simulink model "final_quadruped_230622"  (R2021a)
settings: Solver=ode15s  StartTime=0.0  StopTime=10  FixedStep=1e-3  RelTol=1e-5  EnableMultiTasking=on
values from neighbouring files (symbols this model uses):
  foot_x = 8    [bipedparameters.m]    (also in fcn.m; finalrobotParameters.m; finalrobotParameters_110522.m; finalrobotParameters_140522.m)
  foot_y = 6    [bipedparameters.m]    (also in fcn.m; finalrobotParameters.m; finalrobotParameters_110522.m; finalrobotParameters_140522.m)
  foot_z = 1    [bipedparameters.m]    (also in fcn.m; finalrobotParameters.m; finalrobotParameters_110522.m; finalrobotParameters_140522.m)
  height_plane = 0.025    [bipedparameters.m]    (also in finalrobotParameters.m; finalrobotParameters_110522.m; finalrobotParameters_140522.m; finalrobotParameters_240522.m)
  kd_ankle = 1000    [bipedparameters.m]    (also in finalrobotParameters_240522.m)
  kd_hip = 1000    [bipedparameters.m]    (also in finalrobotParameters_240522.m)
  kd_knee = 1000    [bipedparameters.m]    (also in finalrobotParameters_240522.m)
  ki_ankle = 1000    [bipedparameters.m]    (also in finalrobotParameters_240522.m)
  ki_hip = 1000    [bipedparameters.m]    (also in finalrobotParameters_240522.m)
  ki_knee = 2000    [bipedparameters.m]    (also in finalrobotParameters_240522.m)
  kp_ankle = 1000    [bipedparameters.m]    (also in finalrobotParameters_240522.m)
  kp_hip = 1000    [bipedparameters.m]    (also in finalrobotParameters_240522.m)
  kp_knee = 2000    [bipedparameters.m]    (also in finalrobotParameters_240522.m)
  lower_leg_length = 10    [bipedparameters.m]    (also in fcn.m; finalrobotParameters.m; finalrobotParameters_110522.m; finalrobotParameters_140522.m)
  plane_x = 25    [bipedparameters.m]    (also in finalrobotParameters.m; finalrobotParameters_110522.m; finalrobotParameters_140522.m; finalrobotParameters_240522.m)
  plane_y = 3    [bipedparameters.m]    (also in finalrobotParameters.m; finalrobotParameters_110522.m; finalrobotParameters_140522.m; finalrobotParameters_240522.m)
  torso_offset_x = -0.5    [bipedparameters.m]    (also in finalrobotParameters.m = 10; finalrobotParameters_110522.m = 10; finalrobotParameters_140522.m = 10; finalrobotParameters_240522.m = 10)
  torso_offset_z = -2    [bipedparameters.m]    (also in finalrobotParameters.m; finalrobotParameters_110522.m; finalrobotParameters_140522.m; finalrobotParameters_240522.m)
  torso_x = 5    [bipedparameters.m]    (also in fcn.m = 25; finalrobotParameters.m = 25; finalrobotParameters_110522.m = 25; finalrobotParameters_140522.m = 25)
  torso_y = 10    [bipedparameters.m]    (also in fcn.m = 16; finalrobotParameters.m = 16; finalrobotParameters_110522.m = 16; finalrobotParameters_140522.m = 16)
  torso_z = 8    [bipedparameters.m]    (also in fcn.m = 10; finalrobotParameters.m = 10; finalrobotParameters_110522.m = 10; finalrobotParameters_140522.m = 10)
  upper_leg_length = 10    [bipedparameters.m]    (also in fcn.m; finalrobotParameters.m; finalrobotParameters_110522.m; finalrobotParameters_140522.m)
undefined symbols (not defined in the file or in its folder): sigbuilder_block, X, Y, Z
libraries: nesl_utility x246, sm_lib x71, pid_lib x20, Contact_Forces_Lib x16, fl_lib x4
(part 1 of 8)
settings Model: Creator=Durbadal Guest  LastModifiedBy=Saniya
settings DataIOCC: LimitDataPoints=on  SaveFormat=StructureWithTime  ReturnWorkspaceOutputs=off
settings OptimizationCC: LifeSpan=inf
settings DebuggingCC: SFUnexpectedBacktrackingDiag=warning  SFNoUnconditionalDefaultTransitionDiag=warning  SFExecutionAtInitializationDiag=none  SFMachineParentedDataDiag=warning  ArithmeticOperatorsInVariantConditions=warning
settings HardwareCC: ProdBitPerSizeT=32  ProdBitPerPtrDiffT=32  ProdWordSize=32  ProdHWDeviceType=Specified
settings SFSimCC: SimUseLocalCustomCode=off  CustomCodeUndefinedFunction=UseInterfaceOnly
settings RTWCC: RTWUseLocalCustomCode=off
settings CodeAppCC: StateflowObjectComments=on
settings GRTTargetCC: TargetLangStandard=C89/C90 (ANSI)
settings ConfigComp: CovMetricSettings=dw  CovSaveCumulativeToWorkspaceVar=on  CovSaveSingleToWorkspaceVar=on  CovExternalEMLEnable=off  CovSFcnEnable=off
settings SimscapeCC: SimscapeNominalValues="[{\"value\":\"10\",\"unit\":\"V\"},{\"value\":\"1\",\"unit\":\"A\"},{\"value\":\"10\",\"unit\":\"N*m\"},{\"value\":\"10\",\"unit\":\"bar\"},{\"value\":\"100\",\"unit\":\"kJ/kg\"},{\"value\":\"1\",\"unit\":\"kW\"},{\"value\":\"300\",\"unit\":\"K\"},{\"value\":\"100\",\"unit\":\"cm^3/s\"},{\"value\":\"1\",\"unit\":\"kN\"},{\"value\":\"1\",\"unit\":\"g/cm^3\"},{\"value\":\"1\",\"unit\":\"l\"},{\"value\":\"1\",\"unit\":\"cm^2\"},{\"value\":\"60\",\"unit\":\"Hz\"}]"  SimscapeLogType=all  SimscapeLogDataHistory=10000
settings ConfigurationSet: Description=SimMechanics 2G
settings DiagnosticsConfigSet: SimMechanicsRigidlyBoundBlock=none

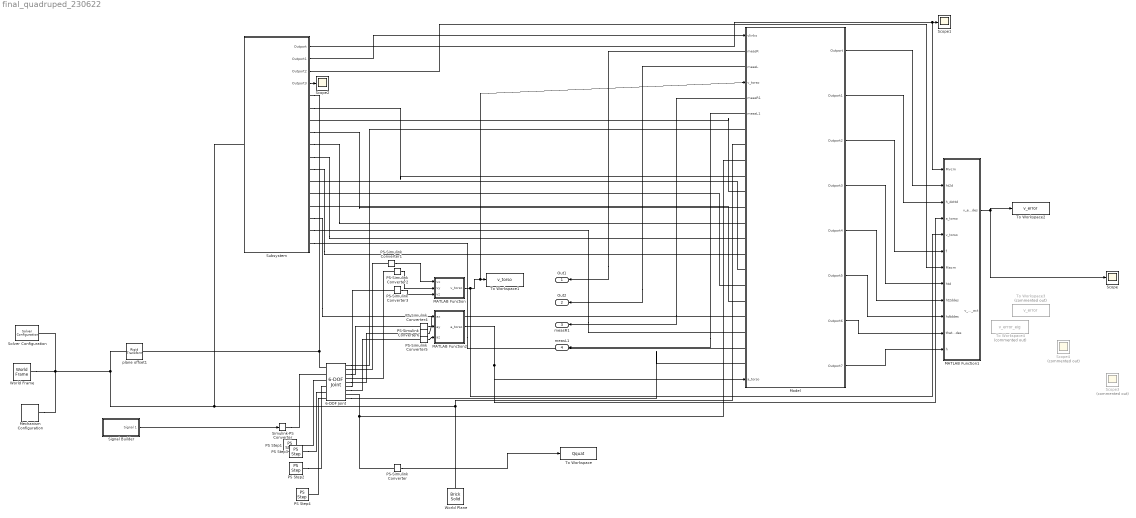
== system final_quadruped_230622 ==
  6-DOF Joint : sm_lib/Joints/6-DOF Joint  JointMode=Normal  SenseConstraintForce=off  SenseConstraintForceX=off  SenseConstraintForceY=off  SenseConstraintForceZ=off  SenseConstraintTorque=off  SenseConstraintTorqueX=off  SenseConstraintTorqueY=off  SenseConstraintTorqueZ=off  SenseTotalForce=off  SenseTotalForceX=off  SenseTotalForceY=off  SenseTotalForceZ=off  SenseTotalTorque=off  SenseTotalTorqueX=off  SenseTotalTorqueY=off  SenseTotalTorqueZ=off  CompositeWrenchDir=FollowerOnBase  CompositeWrenchFrame=BaseFrame  PxEquilibriumPosition=0  PxEquilibriumPositionUnits=m  PxSpringStiffness=0  PxSpringStiffnessUnits=N/m  PxDampingCoefficient=0  PxDampingCoefficientUnits=N/(m/s)  PxTorqueActuationMode=InputTorque  PxMotionActuationMode=ComputedMotion  PxSensePosition=off  PxSenseVelocity=on  PxSenseAcceleration=on  PxSenseTorqueForce=off  PxSenseLowerLimitTorqueForce=off  PxSenseUpperLimitTorqueForce=off  PxLowerLimitSpecify=off  PxLowerLimitBound=-1  PxLowerLimitBoundUnits=m  PxLowerLimitStiffness=1e6  PxLowerLimitStiffnessUnits=N/m  PxLowerLimitDamping=1e3  PxLowerLimitDampingUnits=N/(m/s)  PxLowerLimitTransitionRegionWidth=1e-4  PxLowerLimitTransitionRegionWidthUnits=m  PxUpperLimitSpecify=off  PxUpperLimitBound=1  PxUpperLimitBoundUnits=m  PxUpperLimitStiffness=1e6  PxUpperLimitStiffnessUnits=N/m  PxUpperLimitDamping=1e3  PxUpperLimitDampingUnits=N/(m/s)  PxUpperLimitTransitionRegionWidth=1e-4  PxUpperLimitTransitionRegionWidthUnits=m  PxPositionTargetSpecify=on  PxPositionTargetPriority=High  PxPositionTargetValue=0  PxPositionTargetValueUnits=m  PxVelocityTargetSpecify=off  PxVelocityTargetPriority=High  PxVelocityTargetValue=0  PxVelocityTargetValueUnits=m/s  PyEquilibriumPosition=0  PyEquilibriumPositionUnits=m  PySpringStiffness=0  PySpringStiffnessUnits=N/m  PyDampingCoefficient=0  PyDampingCoefficientUnits=N/(m/s)  PyTorqueActuationMode=InputTorque  PyMotionActuationMode=ComputedMotion  PySensePosition=off  PySenseVelocity=on  PySenseAcceleration=on  PySenseTorqueForce=off  PySenseLowerLimitTorqueForce=off  PySenseUpperLimitTorqueForce=off  PyLowerLimitSpecify=off  PyLowerLimitBound=-1  PyLowerLimitBoundUnits=m  PyLowerLimitStiffness=1e6  PyLowerLimitStiffnessUnits=N/m  PyLowerLimitDamping=1e3  PyLowerLimitDampingUnits=N/(m/s)  PyLowerLimitTransitionRegionWidth=1e-4  PyLowerLimitTransitionRegionWidthUnits=m  PyUpperLimitSpecify=off  PyUpperLimitBound=1  PyUpperLimitBoundUnits=m  PyUpperLimitStiffness=1e6  PyUpperLimitStiffnessUnits=N/m  PyUpperLimitDamping=1e3  PyUpperLimitDampingUnits=N/(m/s)  PyUpperLimitTransitionRegionWidth=1e-4  PyUpperLimitTransitionRegionWidthUnits=m  PyPositionTargetSpecify=on  PyPositionTargetPriority=High  PyPositionTargetValue=0  PyPositionTargetValueUnits=m  PyVelocityTargetSpecify=off  PyVelocityTargetPriority=High  PyVelocityTargetValue=0  PyVelocityTargetValueUnits=m/s  PzEquilibriumPosition=0  PzEquilibriumPositionUnits=m  PzSpringStiffness=0  PzSpringStiffnessUnits=N/m  PzDampingCoefficient=0  PzDampingCoefficientUnits=N/(m/s)  PzTorqueActuationMode=InputTorque  PzMotionActuationMode=ComputedMotion  PzSensePosition=off  PzSenseVelocity=on  PzSenseAcceleration=on  PzSenseTorqueForce=off  PzSenseLowerLimitTorqueForce=off  PzSenseUpperLimitTorqueForce=off  PzLowerLimitSpecify=off  PzLowerLimitBound=-1  PzLowerLimitBoundUnits=m  PzLowerLimitStiffness=1e6  PzLowerLimitStiffnessUnits=N/m  PzLowerLimitDamping=1e3  PzLowerLimitDampingUnits=N/(m/s)  PzLowerLimitTransitionRegionWidth=1e-4  PzLowerLimitTransitionRegionWidthUnits=m  PzUpperLimitSpecify=off  PzUpperLimitBound=1  PzUpperLimitBoundUnits=m  PzUpperLimitStiffness=1e6  PzUpperLimitStiffnessUnits=N/m  PzUpperLimitDamping=1e3  PzUpperLimitDampingUnits=N/(m/s)  PzUpperLimitTransitionRegionWidth=1e-4  PzUpperLimitTransitionRegionWidthUnits=m  PzPositionTargetSpecify=on  PzPositionTargetPriority=High  PzPositionTargetValue=0  PzPositionTargetValueUnits=m  PzVelocityTargetSpecify=off  PzVelocityTargetPriority=High  PzVelocityTargetValue=0  PzVelocityTargetValueUnits=m/s  SphDefPosRotationMethod=None  SphDefPosRotationAngleUnits=deg  SphDefPosRotationStandardAxis=+Z  SphDefPosRotationAngle=0.0  SphDefPosRotationArbitraryAxis=[0 0 1]  SphDefPosFollAlignAxisA=+X  SphDefPosBaseAlignAxisA=+Y  SphDefPosFollAlignAxisB=+Y  SphDefPosBaseAlignAxisB=+Z  SphDefPosRotationSequenceAxes=FollowerAxes  SphDefPosRotationSequence=XYX  SphDefPosRotationSequenceAngles=[0 0 0]  SphDefPosRotationSequenceAnglesUnits=deg  SphDefPosRotationMatrix=[1 0 0; 0 1 0; 0 0 1]  SphEqPosRotationMethod=None  SphEqPosRotationAngleUnits=deg  SphEqPosRotationStandardAxis=+Z  SphEqPosRotationAngle=0.0  SphEqPosRotationArbitraryAxis=[0 0 1]  SphEqPosFollAlignAxisA=+X  SphEqPosBaseAlignAxisA=+Y  SphEqPosFollAlignAxisB=+Y  SphEqPosBaseAlignAxisB=+Z  SphEqPosRotationSequenceAxes=FollowerAxes  SphEqPosRotationSequence=XYX  SphEqPosRotationSequenceAngles=[0 0 0]  SphEqPosRotationSequenceAnglesUnits=deg  SphEqPosRotationMatrix=[1 0 0; 0 1 0; 0 0 1]  SphSpringStiffness=0  SphSpringStiffnessUnits=N*m/deg  SphDampingCoefficient=world_rot_damping  SphDampingCoefficientUnits=N*m/(deg/s)  SphActuateTorqueX=on  SphActuateTorqueY=off  SphActuateTorqueZ=on  SphActuateTorque=off  SphTorqueActuationMode=InputTorque  SphMotionActuationMode=ComputedMotion  SphActuationFrame=BaseFrame  SphSensePosition=on  SphSenseVelocityX=off  SphSenseVelocityY=off  SphSenseVelocityZ=off  SphSenseVelocity=on  SphSenseAccelerationX=off  SphSenseAccelerationY=off  SphSenseAccelerationZ=off  SphSenseAcceleration=off  SphSenseTorqueX=off  SphSenseTorqueY=off  SphSenseTorqueZ=off  SphSenseTorqueForce=off  SphSenseLowerLimitTorqueMag=off  SphSenseUpperLimitTorqueMag=off  SphSensingFrame=BaseFrame  SphLowerLimitSpecify=off  SphLowerLimitBound=15  SphLowerLimitBoundUnits=deg  SphLowerLimitStiffness=1e4  SphLowerLimitStiffnessUnits=N*m/deg  SphLowerLimitDamping=10  SphLowerLimitDampingUnits=N*m/(deg/s)  SphLowerLimitTransitionRegionWidth=0.1  SphLowerLimitTransitionRegionWidthUnits=deg  SphUpperLimitSpecify=off  SphUpperLimitBound=45  SphUpperLimitBoundUnits=deg  SphUpperLimitStiffness=1e4  SphUpperLimitStiffnessUnits=N*m/deg  SphUpperLimitDamping=10  SphUpperLimitDampingUnits=N*m/(deg/s)  SphUpperLimitTransitionRegionWidth=0.1  SphUpperLimitTransitionRegionWidthUnits=deg  SphPositionTargetRotationMethod=None  SphPositionTargetRotationAngleUnits=deg  SphPositionTargetRotationStandardAxis=+Z  SphPositionTargetRotationAngle=0.0  SphPositionTargetRotationArbitraryAxis=[0 0 1]  SphPositionTargetFollAlignAxisA=+X  SphPositionTargetBaseAlignAxisA=+Y  SphPositionTargetFollAlignAxisB=+Y  SphPositionTargetBaseAlignAxisB=+Z  SphPositionTargetRotationSequenceAxes=FollowerAxes  SphPositionTargetRotationSequence=XYX  SphPositionTargetRotationSequenceAngles=[0 0 0]  SphPositionTargetRotationSequenceAnglesUnits=deg  SphPositionTargetRotationMatrix=[1 0 0; 0 1 0; 0 0 1]  SphPositionTargetSpecify=off  SphPositionTargetPriority=High  SphVelocityTargetValue=[0 0 0]  SphVelocityTargetValueUnits=deg/s  SphVelocityTargetSpecify=off  SphVelocityTargetPriority=High  SphVelocityTargetInFollowerFrame=on
  MATLAB Function : MATLAB Function  TreatAsAtomicUnit=on
  MATLAB Function1 : MATLAB Function  TreatAsAtomicUnit=on
  MATLAB Function2 : MATLAB Function  TreatAsAtomicUnit=on
  Mechanism Configuration : sm_lib/Utilities/Mechanism Configuration  UniformGravity=Constant  GravityVector=[0 0 -9.80665]  GravityVectorUnits=m/s^2  GravityUnits=m/s^2  LinearizationDelta=0.001  JointModeTransitionNonlinearIterations=2
  Model : Subsystem
      settings: PortSchema="{\"entries\":[{\"content\":{\"sides\":[{\"content\":{\"connectorIds\":[\"Out5\",\"Out6\",\"Out7\",\"Out8\",\"Out9\",\"Out10\",\"Out11\",\"Out12\"]},\"type\":\"ConnectorPlacement.EquallySpacedRectSide\",\"uuid\":\"648e0f1c-94fd-432d-b314-f859853b28dc\"},{\"content\":{\"connectorIds\":[\"In1\",\"Out1\",\"Out2\",\"In2\",\"Out3\",\"Out4\",\"RConn1\",\"RConn2\",\"RConn3\",\"RConn4\",\"RConn5\",\"RConn6\",\"RConn7\",\"RConn8\",\"RConn9\",\"RConn10\",\"RConn11\",\"RConn12\",\"RConn13\",\"RConn14\",\"RConn15\",\"RConn16\",\"In3\"],\"side\":\"RIGHT\"},\"type\":\"ConnectorPlacement.EquallySpacedRectSide\",\"uuid\":\"4a085109-6c7b-452e-9c34-33db191f9143\"},{\"content\":{\"connectorIds\":[],\"side\":\"TOP\"},\"type\":\"ConnectorPlacement.EquallySpacedRectSide\",\"uuid\":\"a578f37e-fb06-4d5d-8e21-8bc1ba433708\"},{\"content\":{\"connectorIds\":[],\"side\":\"BOTTOM\"},\"type\":\"ConnectorPlacement.EquallySpacedRectSide\",\"uuid\":\"167a25d4-eaf5-4df2-a71c-c676bae0267f\"}]},\"type\":\"ConnectorPlacement.EquallySpacedConnector\",\"uuid\":\"512c293d-fddc-4597-a716-0ff05cc0aa2f\"}],\"packageUris\":[\"http://schema.mathworks.com/mf0/Connector/R2020b\"],\"version\":\"1.0\"}"
  PS Step1 : fl_lib/Physical Signals/Sources/PS Step  step_time=0 s  initial_value=0 N  final_value=0 N
      settings: SourceProductBaseCode=SS
  PS Step2 : fl_lib/Physical Signals/Sources/PS Step  step_time=1 s  initial_value=0 N  final_value=0 N
      settings: SourceProductBaseCode=SS
  PS Step3 : fl_lib/Physical Signals/Sources/PS Step  step_time=1 s  initial_value=0 N*m  final_value=0 N*m
      settings: SourceProductBaseCode=SS
  PS Step4 : fl_lib/Physical Signals/Sources/PS Step  step_time=0 s  initial_value=0 N*m  final_value=1 N*m
      settings: SourceProductBaseCode=SS
  PS-Simulink Converter{,1..6} (7 alike) : nesl_utility/PS-Simulink Converter  PhysicalDomain=network_engine_domain  SubClassName=ps_output  LeftPortType=input  RightPortType=output  PseudoPeriodic=off  Frequencies=[]  Unit=inherit  AffineConversion=off
      settings: SourceProductBaseCode=PW,SS
  Scope : Scope
  Scope1 : Scope
  Scope2 : Scope
  Scope3 : Scope  Commented=on
  Scope4 : Scope  Commented=on
  Signal Builder : Subsystem  Tag=STV Subsys  LoadFcn=sigbuilder_block('load');  StartFcn=sigbuilder_block('start');  StopFcn=sigbuilder_block('stop');  ClipboardFcn=sigbuilder_block('clipboard');  mask(Sigbuilder block){tuvar=[0:10]}
      mask help: Simulink:masks:SigbuilderBlock_MD
      mask init:
      | if ~strcmp(get_param(bdroot(gcbh),'SimulationStatus'),'stopped') tuvar = sigbuilder_block('maskInit'); end
      settings: CopyFcn=sigbuilder_block('copy');  DeleteFcn=sigbuilder_block('delete');  ModelCloseFcn=sigbuilder_block('modelClose');  PreSaveFcn=sigbuilder_block('preSave');  PauseFcn=sigbuilder_block('pause');  ContinueFcn=sigbuilder_block('continue');  NameChangeFcn=sigbuilder_block('namechange');  OpenFcn=sigbuilder_block('open',[5.5 36 949 412 ]);  CloseFcn=sigbuilder_block('close');
      mask Display: plot(0, 0, 100, 100,[2, 2, 32, 32, 2], [68, 8, 8, 68, 68],[32, 2], [38, 38], [32, 19, 2],[53, 60, 44], [32, 17, 17, 2],[16, 16, 31, 31]);txt = getActiveGroup(gcbh);text(2, 100, txt,'verticalAlignment', 'top');
  Simulink-PS Converter : nesl_utility/Simulink-PS Converter  PhysicalDomain=network_engine_domain  SubClassName=ps_input  LeftPortType=input  RightPortType=output  PseudoPeriodic=off  Frequencies=[]  NoiseDistribution=none  NoiseParameters=[]  Unit=1  AffineConversion=off  FilteringAndDerivatives=provide  SimscapeFilterOrder=1  InputFilterTimeConstant=0.001  UdotUserProvided=0
      settings: SourceProductBaseCode=PW,SS
  Solver Configuration : nesl_utility/Solver Configuration  PhysicalDomain=network_engine_domain  SubClassName=solver  LeftPortType=input  RightPortType=generic  Tones=[]  Harmonics=[]  SimulateNoise=off  Profile=off  UseLocalSampling=off  EnableSwitchedLinearOptims=on  FrequencyDomain=off  UseCCode=off  RelTol=0.001  AbsTol=1e-06  MinStep=1e-09  ToWorkspace=off  RevertToSquareIcSolve=off  NumHomotopyIterations=100  PhasorMode=off  PhasorModeNumHarmonics=1  DoDC=off  ResidualTolerance=1e-09  UseLocalSolver=off  LocalSolverChoice=NE_BACKWARD_EULER_ADVANCER  LocalSolverSampleTime=0.001  DoFixedCost=off  MaxNonlinIter=3  MaxModeIter=2  ComputeImpulses=off  ImpulseIterations=2  LinearAlgebra=Full  EquationFormulation=NE_TIME_EF  DelaysMemoryBudget=1024  AutomaticFiltering=on  FilteringTimeConstant=0.001  PartitionStorageMethod=AS_NEEDED  PartitionMemoryBudget=1024  PartitionMethod=FAST
      settings: SourceProductBaseCode=PW,SS
  Subsystem : Subsystem
  To Workspace : ToWorkspace  VariableName=Qquat  SaveFormat=Timeseries  SampleTime=-1
  To Workspace1 : ToWorkspace  VariableName=v_torso  SaveFormat=Timeseries  SampleTime=-1
  To Workspace2 : ToWorkspace  VariableName=v_error  SaveFormat=Timeseries  SampleTime=-1
  To Workspace3 : ToWorkspace  Commented=on  VariableName=v_error  SaveFormat=Timeseries  SampleTime=-1
  To Workspace4 : ToWorkspace  Commented=on  VariableName=v_error_eig  SaveFormat=Timeseries  SampleTime=-1
  World Frame : sm_lib/Frames and Transforms/World Frame
  World Plane : sm_lib/Body Elements/Brick Solid  GraphicAmbientColor=[0.15 0.15 0.15 1.0]  BasedOnType=Density  BrickDimensions=[plane_x plane_y height_plane]  BrickDimensionUnits=m  CenterOfMass=[0 0 0]  CenterOfMassUnits=m  GraphicDiffuseColor=[1.0 0.2 0.2]  Density=2000  DensityUnits=kg/m^3  DoExposeReferenceFrame=on  GraphicEmissiveColor=[0.0 0.0 0.0 1.0]  ExportEntireGeometry=off  SerializedFrames=<Frames/>  MarkerShape=Sphere  MarkerSize=10  GraphicType=FromGeometry  InertiaType=CalculateFromGeometry  Mass=1  MassUnits=kg  MomentsOfInertia=[1 1 1]  MomentsOfInertiaUnits=kg*m^2  GraphicOpacity=1.0  ProductsOfInertia=[1 1 1]  ProductsOfInertiaUnits=kg*m^2  GraphicShininess=75  GraphicSpecularColor=[0.5 0.5 0.5 1.0]  GraphicVisPropType=SimpleVisualProperties
  plane offset1 : sm_lib/Frames and Transforms/Rigid Transform  TranslationMethod=StandardAxis  TranslationStandardOffset=24.1  TranslationLengthUnit=cm  TranslationStandardAxis=+Z  TranslationCartesianOffset=[0 0 0]  TranslationROffset=0  TranslationROffsetUnits=m  TranslationZOffset=0  TranslationZOffsetUnits=m  TranslationThetaOffset=0  TranslationThetaOffsetUnits=deg  RotationMethod=None  RotationAngleUnits=deg  RotationStandardAxis=+Z  RotationAngle=0.0  RotationArbitraryAxis=[0 0 1]  FollAlignAxisA=+X  BaseAlignAxisA=+Y  FollAlignAxisB=+Y  BaseAlignAxisB=+Z  RotationSequenceAxes=FollowerAxes  RotationSequence=XYX  RotationSequenceAngles=[0 0 0]  RotationSequenceAnglesUnits=deg  RotationMatrix=[1 0 0; 0 1 0; 0 0 1]
  Out1 : Outport  VectorParamsAs1DForOutWhenUnconnected=off
  Out2 : Outport  Port=2  VectorParamsAs1DForOutWhenUnconnected=off
  measR1 : Outport  Port=3  VectorParamsAs1DForOutWhenUnconnected=off
  measL1 : Outport  Port=4  VectorParamsAs1DForOutWhenUnconnected=off
  wires:
  Model/1(measR) -> Out1/1
  Model/2(measL) -> Out2/1
  Model/3(measR1) -> measR1/1
  Model/4(measL1) -> measL1/1
  PS-Simulink Converter/1 -> To Workspace/1
  PS-Simulink Converter1/1 -> MATLAB Function/1(vx)
  PS-Simulink Converter2/1 -> MATLAB Function/2(vy)
  PS-Simulink Converter3/1 -> MATLAB Function/3(vz)
  Subsystem/1(Outport) -> Scope1/1, MATLAB Function1/1(Mvcm)
  Model/5(Outport) -> MATLAB Function1/2(ht2d)
  MATLAB Function/1(v_torso) -> MATLAB Function1/5(v_torso), To Workspace1/1, Model/2(v_torso)
  Subsystem/2(Outport1) -> Model/1(vlinks)
  PS-Simulink Converter4/1 -> MATLAB Function2/1(ax)
  PS-Simulink Converter5/1 -> MATLAB Function2/3(az)
  PS-Simulink Converter6/1 -> MATLAB Function2/2(ay)
  MATLAB Function2/1(a_torso) -> MATLAB Function1/4(a_torso), Model/3(a_torso)
  Model/6(Outport1) -> MATLAB Function1/3(h_dottd)
  Model/7(Outport2) -> MATLAB Function1/6(f)
  Subsystem/3(Outport2) -> MATLAB Function1/7(Macm)
  Subsystem/4(Outport3) -> Scope2/1
  Model/8(Outport3) -> MATLAB Function1/8(htd)
  MATLAB Function1/1(v_error_des) -> Scope/1, To Workspace2/1
  Model/9(Outport4) -> MATLAB Function1/9(ht2ddes)
  Model/10(Outport5) -> MATLAB Function1/10(hdtddes)
  ? -> Scope3/1, To Workspace3/1
  Model/11(Outport6) -> MATLAB Function1/11(theta_d_des)
  Model/12(Outport7) -> MATLAB Function1/12(h)
  ? -> Scope4/1, To Workspace4/1
  Signal Builder/1(Signal 1) -> Simulink-PS Converter/1
  connections:
  6-DOF Joint/RConn1 -- Model/RConn1
  6-DOF Joint/LConn1 -- plane offset1/RConn1 -- Subsystem/RConn1
  PS-Simulink Converter/LConn1 -- 6-DOF Joint/RConn8 -- Model/RConn3
  PS-Simulink Converter1/LConn1 -- 6-DOF Joint/RConn2
  PS-Simulink Converter2/LConn1 -- 6-DOF Joint/RConn4
  plane offset1/LConn1 -- Solver Configuration/RConn1 -- World Frame/RConn1 -- Mechanism Configuration/RConn1 -- Subsystem/LConn1 -- World Plane/RConn1 -- Model/RConn2
  Subsystem/RConn2 -- Model/RConn4
  Model/RConn5 -- Subsystem/RConn3
  Subsystem/RConn4 -- Model/RConn6
  Subsystem/RConn5 -- Model/RConn7
  Subsystem/RConn6 -- Model/RConn8
  Subsystem/RConn7 -- Model/RConn9
  Model/RConn10 -- Subsystem/RConn8
  Model/RConn11 -- Subsystem/RConn9
  Model/RConn12 -- Subsystem/RConn10
  Subsystem/RConn11 -- Model/RConn13
  Subsystem/RConn12 -- Model/RConn14
  Subsystem/RConn13 -- Model/RConn15
  PS Step1/RConn1 -- 6-DOF Joint/LConn3
  PS Step2/RConn1 -- 6-DOF Joint/LConn4
  PS Step3/RConn1 -- 6-DOF Joint/LConn5
  6-DOF Joint/RConn9 -- Model/RConn16
  6-DOF Joint/RConn6 -- PS-Simulink Converter3/LConn1
  6-DOF Joint/RConn3 -- PS-Simulink Converter4/LConn1
  6-DOF Joint/RConn5 -- PS-Simulink Converter6/LConn1
  6-DOF Joint/RConn7 -- PS-Simulink Converter5/LConn1
  Simulink-PS Converter/RConn1 -- 6-DOF Joint/LConn2
  6-DOF Joint/LConn6 -- PS Step4/RConn1

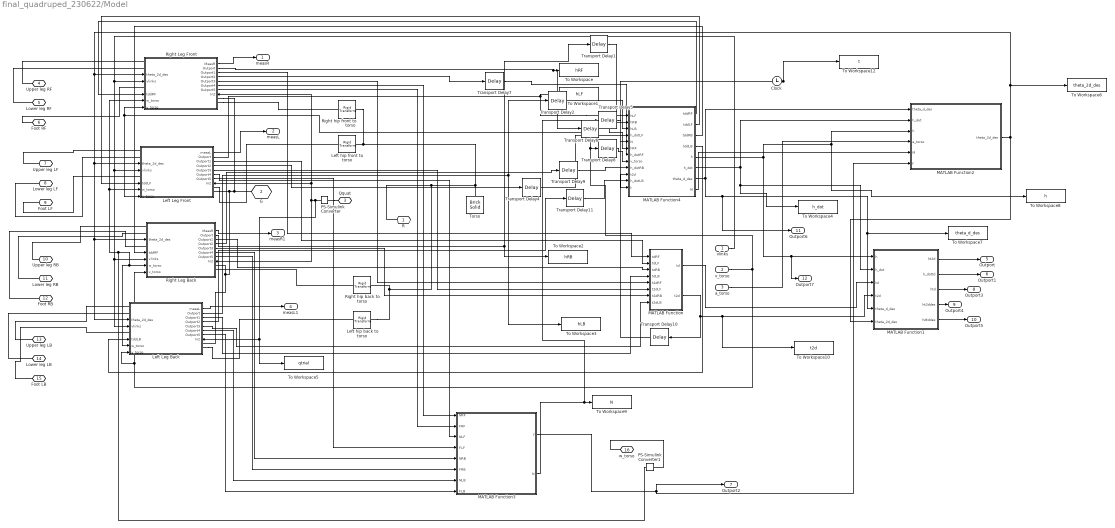
== system final_quadruped_230622/Model ==
  vlinks : Inport
  v_torso : Inport  Port=2
  a_torso : Inport  Port=3
  Clock : Clock
  Left Leg Back : Subsystem
      settings: PortSchema="{\"entries\":[{\"content\":{\"sides\":[{\"content\":{\"connectorIds\":[\"LConn1\",\"LConn2\",\"In1\",\"In2\",\"LConn3\",\"In3\",\"In4\",\"In5\"]},\"type\":\"ConnectorPlacement.EquallySpacedRectSide\",\"uuid\":\"22ee734e-d516-4767-9dd7-a84a6d7499a1\"},{\"content\":{\"connectorIds\":[\"Out1\",\"Out2\",\"Out3\",\"Out4\",\"Out5\",\"Out6\",\"Out7\",\"In6\",\"RConn1\",\"RConn2\"],\"side\":\"RIGHT\"},\"type\":\"ConnectorPlacement.EquallySpacedRectSide\",\"uuid\":\"10c942f7-94ea-46a3-ba7f-65e81ae36ff4\"},{\"content\":{\"connectorIds\":[],\"side\":\"TOP\"},\"type\":\"ConnectorPlacement.EquallySpacedRectSide\",\"uuid\":\"f15406a8-c456-4a24-8e06-fd295582a32c\"}]},\"type\":\"ConnectorPlacement.EquallySpacedConnector\",\"uuid\":\"8882591f-f267-4868-b883-a2707b6c50ed\"}],\"packageUris\":[\"http://schema.mathworks.com/mf0/Connector/R2020b\"],\"version\":\"1.0\"}"
  "Left Leg Front " : Subsystem
      settings: PortSchema="{\"entries\":[{\"content\":{\"sides\":[{\"content\":{\"connectorIds\":[\"LConn1\",\"LConn2\",\"In1\",\"In2\",\"LConn3\",\"In3\",\"In4\",\"In5\"]},\"type\":\"ConnectorPlacement.EquallySpacedRectSide\",\"uuid\":\"22ee734e-d516-4767-9dd7-a84a6d7499a1\"},{\"content\":{\"connectorIds\":[\"Out1\",\"Out2\",\"Out3\",\"Out4\",\"Out5\",\"Out6\",\"Out7\",\"In6\",\"RConn1\",\"RConn2\"],\"side\":\"RIGHT\"},\"type\":\"ConnectorPlacement.EquallySpacedRectSide\",\"uuid\":\"10c942f7-94ea-46a3-ba7f-65e81ae36ff4\"},{\"content\":{\"connectorIds\":[],\"side\":\"TOP\"},\"type\":\"ConnectorPlacement.EquallySpacedRectSide\",\"uuid\":\"f15406a8-c456-4a24-8e06-fd295582a32c\"}]},\"type\":\"ConnectorPlacement.EquallySpacedConnector\",\"uuid\":\"8882591f-f267-4868-b883-a2707b6c50ed\"}],\"packageUris\":[\"http://schema.mathworks.com/mf0/Connector/R2020b\"],\"version\":\"1.0\"}"
  Left hip back to torso : sm_lib/Frames and Transforms/Rigid Transform  TranslationMethod=Cartesian  TranslationStandardOffset=0  TranslationLengthUnit=cm  TranslationStandardAxis=+Z  TranslationCartesianOffset=[-torso_offset_x torso_y/2 torso_offset_z]  TranslationROffset=0  TranslationROffsetUnits=m  TranslationZOffset=0  TranslationZOffsetUnits=m  TranslationThetaOffset=0  TranslationThetaOffsetUnits=deg  RotationMethod=None  RotationAngleUnits=deg  RotationStandardAxis=+Z  RotationAngle=0.0  RotationArbitraryAxis=[0 0 1]  FollAlignAxisA=+X  BaseAlignAxisA=+Y  FollAlignAxisB=+Y  BaseAlignAxisB=+Z  RotationSequenceAxes=FollowerAxes  RotationSequence=XYX  RotationSequenceAngles=[0 0 0]  RotationSequenceAnglesUnits=deg  RotationMatrix=[1 0 0; 0 1 0; 0 0 1]
  Left hip front to torso : sm_lib/Frames and Transforms/Rigid Transform  TranslationMethod=Cartesian  TranslationStandardOffset=0  TranslationLengthUnit=cm  TranslationStandardAxis=+Z  TranslationCartesianOffset=[torso_offset_x torso_y/2 torso_offset_z]  TranslationROffset=0  TranslationROffsetUnits=m  TranslationZOffset=0  TranslationZOffsetUnits=m  TranslationThetaOffset=0  TranslationThetaOffsetUnits=deg  RotationMethod=None  RotationAngleUnits=deg  RotationStandardAxis=+Z  RotationAngle=0.0  RotationArbitraryAxis=[0 0 1]  FollAlignAxisA=+X  BaseAlignAxisA=+Y  FollAlignAxisB=+Y  BaseAlignAxisB=+Z  RotationSequenceAxes=FollowerAxes  RotationSequence=XYX  RotationSequenceAngles=[0 0 0]  RotationSequenceAnglesUnits=deg  RotationMatrix=[1 0 0; 0 1 0; 0 0 1]
  MATLAB Function : MATLAB Function  TreatAsAtomicUnit=on
  MATLAB Function1 : MATLAB Function  TreatAsAtomicUnit=on
  MATLAB Function2 : MATLAB Function  TreatAsAtomicUnit=on
  MATLAB Function3 : MATLAB Function  TreatAsAtomicUnit=on
  MATLAB Function4 : MATLAB Function  TreatAsAtomicUnit=on
  PS-Simulink Converter : nesl_utility/PS-Simulink Converter  PhysicalDomain=network_engine_domain  SubClassName=ps_output  LeftPortType=input  RightPortType=output  PseudoPeriodic=off  Frequencies=[]  Unit=inherit  AffineConversion=off
      settings: SourceProductBaseCode=PW,SS
  PS-Simulink Converter1 : nesl_utility/PS-Simulink Converter  PhysicalDomain=network_engine_domain  SubClassName=ps_output  LeftPortType=input  RightPortType=output  PseudoPeriodic=off  Frequencies=[]  Unit=inherit  AffineConversion=off
      settings: SourceProductBaseCode=PW,SS
  Right Leg Back : Subsystem
      settings: PortSchema="{\"entries\":[{\"content\":{\"sides\":[{\"content\":{\"connectorIds\":[\"LConn1\",\"LConn2\",\"In1\",\"LConn3\",\"In2\",\"In3\",\"In4\",\"In5\"]},\"type\":\"ConnectorPlacement.EquallySpacedRectSide\",\"uuid\":\"22ee734e-d516-4767-9dd7-a84a6d7499a1\"},{\"content\":{\"connectorIds\":[\"Out1\",\"Out2\",\"Out3\",\"Out4\",\"Out5\",\"Out6\",\"Out7\",\"In6\",\"RConn1\",\"RConn2\"],\"side\":\"RIGHT\"},\"type\":\"ConnectorPlacement.EquallySpacedRectSide\",\"uuid\":\"10c942f7-94ea-46a3-ba7f-65e81ae36ff4\"},{\"content\":{\"connectorIds\":[],\"side\":\"TOP\"},\"type\":\"ConnectorPlacement.EquallySpacedRectSide\",\"uuid\":\"f15406a8-c456-4a24-8e06-fd295582a32c\"}]},\"type\":\"ConnectorPlacement.EquallySpacedConnector\",\"uuid\":\"8882591f-f267-4868-b883-a2707b6c50ed\"}],\"packageUris\":[\"http://schema.mathworks.com/mf0/Connector/R2020b\"],\"version\":\"1.0\"}"
  "Right Leg Front " : Subsystem
      settings: PortSchema="{\"entries\":[{\"content\":{\"sides\":[{\"content\":{\"connectorIds\":[\"LConn1\",\"LConn2\",\"In1\",\"In2\",\"LConn3\",\"In3\",\"In4\",\"In5\"]},\"type\":\"ConnectorPlacement.EquallySpacedRectSide\",\"uuid\":\"22ee734e-d516-4767-9dd7-a84a6d7499a1\"},{\"content\":{\"connectorIds\":[\"Out1\",\"Out2\",\"Out3\",\"Out4\",\"Out5\",\"Out6\",\"Out7\",\"In6\",\"RConn1\",\"RConn2\"],\"side\":\"RIGHT\"},\"type\":\"ConnectorPlacement.EquallySpacedRectSide\",\"uuid\":\"10c942f7-94ea-46a3-ba7f-65e81ae36ff4\"},{\"content\":{\"connectorIds\":[],\"side\":\"TOP\"},\"type\":\"ConnectorPlacement.EquallySpacedRectSide\",\"uuid\":\"f15406a8-c456-4a24-8e06-fd295582a32c\"}]},\"type\":\"ConnectorPlacement.EquallySpacedConnector\",\"uuid\":\"8882591f-f267-4868-b883-a2707b6c50ed\"}],\"packageUris\":[\"http://schema.mathworks.com/mf0/Connector/R2020b\"],\"version\":\"1.0\"}"
  Right hip back to torso : sm_lib/Frames and Transforms/Rigid Transform  TranslationMethod=Cartesian  TranslationStandardOffset=0  TranslationLengthUnit=cm  TranslationStandardAxis=+Z  TranslationCartesianOffset=[-torso_offset_x -torso_y/2 torso_offset_z]  TranslationROffset=0  TranslationROffsetUnits=m  TranslationZOffset=0  TranslationZOffsetUnits=m  TranslationThetaOffset=0  TranslationThetaOffsetUnits=deg  RotationMethod=None  RotationAngleUnits=deg  RotationStandardAxis=+Z  RotationAngle=0.0  RotationArbitraryAxis=[0 0 1]  FollAlignAxisA=+X  BaseAlignAxisA=+Y  FollAlignAxisB=+Y  BaseAlignAxisB=+Z  RotationSequenceAxes=FollowerAxes  RotationSequence=XYX  RotationSequenceAngles=[0 0 0]  RotationSequenceAnglesUnits=deg  RotationMatrix=[1 0 0; 0 1 0; 0 0 1]
  Right hip front to torso : sm_lib/Frames and Transforms/Rigid Transform  TranslationMethod=Cartesian  TranslationStandardOffset=0  TranslationLengthUnit=cm  TranslationStandardAxis=+Z  TranslationCartesianOffset=[torso_offset_x -torso_y/2 torso_offset_z]  TranslationROffset=0  TranslationROffsetUnits=m  TranslationZOffset=0  TranslationZOffsetUnits=m  TranslationThetaOffset=0  TranslationThetaOffsetUnits=deg  RotationMethod=None  RotationAngleUnits=deg  RotationStandardAxis=+Z  RotationAngle=0.0  RotationArbitraryAxis=[0 0 1]  FollAlignAxisA=+X  BaseAlignAxisA=+Y  FollAlignAxisB=+Y  BaseAlignAxisB=+Z  RotationSequenceAxes=FollowerAxes  RotationSequence=XYX  RotationSequenceAngles=[0 0 0]  RotationSequenceAnglesUnits=deg  RotationMatrix=[1 0 0; 0 1 0; 0 0 1]
  To Workspace : ToWorkspace  VariableName=hRF  SaveFormat=Timeseries  SampleTime=-1
  To Workspace1 : ToWorkspace  VariableName=hLF  SaveFormat=Timeseries  SampleTime=-1
  To Workspace10 : ToWorkspace  VariableName=t2d  SaveFormat=Timeseries  SampleTime=-1
  To Workspace12 : ToWorkspace  VariableName=t  SaveFormat=Timeseries  SampleTime=-1
  To Workspace2 : ToWorkspace  VariableName=hRB  SaveFormat=Timeseries  SampleTime=-1
  To Workspace3 : ToWorkspace  VariableName=hLB  SaveFormat=Timeseries  SampleTime=-1
  To Workspace4 : ToWorkspace  VariableName=h_dot  SaveFormat=Timeseries  SampleTime=-1
  To Workspace5 : ToWorkspace  VariableName=qtrial  SaveFormat=Timeseries  SampleTime=-1
  To Workspace6 : ToWorkspace  VariableName=theta_2d_des  SaveFormat=Timeseries  SampleTime=-1
  To Workspace7 : ToWorkspace  VariableName=theta_d_des  SaveFormat=Timeseries  SampleTime=-1
  To Workspace8 : ToWorkspace  VariableName=h  SaveFormat=Timeseries  SampleTime=-1
  To Workspace9 : ToWorkspace  VariableName=N  SaveFormat=Timeseries  SampleTime=-1
  Torso : sm_lib/Body Elements/Brick Solid  GraphicAmbientColor=[0.15 0.15 0.15 1.0]  BasedOnType=Density  BrickDimensions=[torso_x torso_y torso_z]  BrickDimensionUnits=cm  CenterOfMass=[0 0 0]  CenterOfMassUnits=m  GraphicDiffuseColor=[0.5 0.5 0.5]  Density=1000  DensityUnits=kg/m^3  DoExposeReferenceFrame=on  GraphicEmissiveColor=[0.0 0.0 0.0 1.0]  ExportEntireGeometry=off  SerializedFrames=<Frames/>  MarkerShape=Sphere  MarkerSize=10  GraphicType=FromGeometry  InertiaType=CalculateFromGeometry  Mass=1  MassUnits=kg  MomentsOfInertia=[1 1 1]  MomentsOfInertiaUnits=kg*m^2  GraphicOpacity=1.0  ProductsOfInertia=[1 1 1]  ProductsOfInertiaUnits=kg*m^2  GraphicShininess=75  GraphicSpecularColor=[0.5 0.5 0.5 1.0]  GraphicVisPropType=SimpleVisualProperties
  Transport Delay{1..2,4..11} (10 alike) : TransportDelay  DelayTime=0.0001
  R : PMIOPort  Side=Right
  G : PMIOPort  Port=2  Side=Right
  Qquat : PMIOPort  Port=3  Side=Right
  Upper leg RF : PMIOPort  Port=4  Side=Right
  Lower leg RF : PMIOPort  Port=5  Side=Right
  Foot RF : PMIOPort  Port=6  Side=Right
  Upper leg LF : PMIOPort  Port=7  Side=Right
  Lower leg LF : PMIOPort  Port=8  Side=Right
  Foot LF : PMIOPort  Port=9  Side=Right
  Upper leg RB : PMIOPort  Port=10  Side=Right
  Lower leg RB : PMIOPort  Port=11  Side=Right
  Foot RB : PMIOPort  Port=12  Side=Right
  Upper leg LB : PMIOPort  Port=13  Side=Right
  Lower leg LB : PMIOPort  Port=14  Side=Right
  Foot LB : PMIOPort  Port=15  Side=Right
  w_torso : PMIOPort  Port=16  Side=Right
  measR : Outport  VectorParamsAs1DForOutWhenUnconnected=off
  measL : Outport  Port=2  VectorParamsAs1DForOutWhenUnconnected=off
  measR1 : Outport  Port=3  VectorParamsAs1DForOutWhenUnconnected=off
  measL1 : Outport  Port=4  VectorParamsAs1DForOutWhenUnconnected=off
  Outport : Outport  Port=5
  Outport1 : Outport  Port=6
  Outport2 : Outport  Port=7
  Outport3 : Outport  Port=8
  Outport4 : Outport  Port=9
  Outport5 : Outport  Port=10
  Outport6 : Outport  Port=11
  Outport7 : Outport  Port=12
  wires:
  "Left Leg Front "/1(measL) -> measL/1
  "Right Leg Front "/1(MeasR) -> measR/1
  Right Leg Back/1(MeasR) -> measR1/1
  Left Leg Back/1(measL) -> measL1/1
  "Right Leg Front "/2(Outport) -> Transport Delay6/1, To Workspace/1
  Right Leg Back/2(Outport) -> Transport Delay1/1, To Workspace2/1
  Left Leg Back/2(Outport) -> To Workspace3/1, Transport Delay2/1
  PS-Simulink Converter/1 -> Right Leg Back/6(In2), "Right Leg Front "/6(In2), "Left Leg Front "/6(In2), To Workspace5/1, Left Leg Back/6(In2)
  MATLAB Function4/1(tddRF) -> "Right Leg Front "/3(tddRF)
  MATLAB Function4/2(tddLF) -> "Left Leg Front "/3(tddLF)
  MATLAB Function4/3(tddRB) -> Right Leg Back/2(tddRF)
  MATLAB Function4/4(tddLB) -> Left Leg Back/3(tddLB)
  "Right Leg Front "/3(Outport1) -> MATLAB Function/1(tdRF)
  "Left Leg Front "/3(Outport1) -> MATLAB Function/2(tdLF)
  Right Leg Back/3(Outport1) -> MATLAB Function/3(tdRB)
  Left Leg Back/3(Outport1) -> MATLAB Function/4(tdLB)
  MATLAB Function4/5(h) -> Outport7/1, MATLAB Function1/1(h), To Workspace8/1, MATLAB Function2/3(h)
  MATLAB Function/1(td) -> MATLAB Function1/3(td)
  MATLAB Function1/1(ht2d) -> Outport/1
  v_torso/1 -> "Left Leg Front "/5(v_torso), "Right Leg Front "/5(v_torso), Transport Delay8/1, Right Leg Back/5(v_torso), Left Leg Back/5(v_torso)
  vlinks/1 -> Left Leg Back/2(vlinks), Right Leg Back/3(vlinks), "Left Leg Front "/2(vlinks), "Right Leg Front "/2(vlinks)
  PS-Simulink Converter1/1 -> Left Leg Back/4(w_torso), Right Leg Back/4(w_torso), "Right Leg Front "/4(w_torso), "Left Leg Front "/4(w_torso)
  "Right Leg Front "/4(Outport2) -> Transport Delay7/1
  MATLAB Function4/6(h_dot) -> MATLAB Function2/2(h_dot), MATLAB Function1/2(h_dot), To Workspace4/1
  Right Leg Back/4(Outport2) -> Transport Delay9/1
  Left Leg Back/4(Outport2) -> Transport Delay11/1
  "Right Leg Front "/5(Outport3) -> MATLAB Function/5(t2dRF)
  MATLAB Function4/7(theta_d_des) -> MATLAB Function2/1(theta_d_des), Outport6/1, To Workspace7/1, MATLAB Function1/5(theta_d_des)
  a_torso/1 -> MATLAB Function2/4(a_torso)
  MATLAB Function4/8(M) -> MATLAB Function2/5(M)
  MATLAB Function3/1(f) -> Outport2/1, MATLAB Function2/6(f)
  "Right Leg Front "/6(Outport4) -> MATLAB Function3/1(NRF)
  "Right Leg Front "/7(Outport5) -> MATLAB Function3/2(FRF)
  "Left Leg Front "/6(Outport4) -> MATLAB Function3/3(NLF)
  "Left Leg Front "/7(Outport5) -> MATLAB Function3/4(FLF)
  Right Leg Back/6(Outport4) -> MATLAB Function3/5(NRB)
  Right Leg Back/7(Outport5) -> MATLAB Function3/6(FRB)
  Left Leg Back/7(Outport5) -> MATLAB Function3/8(FLB)
  MATLAB Function2/1(theta_2d_des) -> Left Leg Back/1(theta_2d_des), Right Leg Back/1(theta_2d_des), "Left Leg Front "/1(theta_2d_des), "Right Leg Front "/1(theta_2d_des), To Workspace6/1, MATLAB Function1/6(theta_2d_des)
  Left Leg Back/6(Outport4) -> MATLAB Function3/7(NLB)
  "Left Leg Front "/5(Outport3) -> MATLAB Function/6(t2dLF)
  Right Leg Back/5(Outport3) -> MATLAB Function/7(t2dRB)
  Left Leg Back/5(Outport3) -> MATLAB Function/8(t2dLB)
  MATLAB Function/2(t2d) -> To Workspace10/1, MATLAB Function1/4(t2d), Transport Delay10/1
  MATLAB Function1/2(h_dottd) -> Outport1/1
  MATLAB Function1/3(htd) -> Outport3/1
  MATLAB Function1/4(ht2ddes) -> Outport4/1
  MATLAB Function1/5(hdtddes) -> Outport5/1
  MATLAB Function3/2(N) -> Transport Delay5/1, To Workspace9/1
  "Left Leg Front "/2(Outport) -> MATLAB Function4/1(hLF), To Workspace1/1
  Transport Delay1/1 -> MATLAB Function4/2(hRB)
  Transport Delay2/1 -> MATLAB Function4/3(hLB)
  "Left Leg Front "/4(Outport2) -> Transport Delay4/1
  Transport Delay4/1 -> MATLAB Function4/4(h_dotLF)
  Transport Delay5/1 -> MATLAB Function4/5(N)
  Transport Delay6/1 -> MATLAB Function4/6(hRF)
  Transport Delay7/1 -> MATLAB Function4/7(h_dotRF)
  Transport Delay8/1 -> MATLAB Function4/8(v_torso)
  Transport Delay9/1 -> MATLAB Function4/9(h_dotRB)
  Transport Delay10/1 -> MATLAB Function4/10(t2d)
  Transport Delay11/1 -> MATLAB Function4/11(h_dotLB)
  Clock/1 -> To Workspace12/1, MATLAB Function4/12(t)
  connections:
  Left hip front to torso/RConn1 -- "Left Leg Front "/RConn2
  "Right Leg Front "/RConn2 -- Right hip front to torso/RConn1
  "Right Leg Front "/RConn1 -- "Left Leg Front "/RConn1 -- Left Leg Back/RConn1 -- Right Leg Back/RConn1 -- G/RConn1
  Right hip back to torso/RConn1 -- Right Leg Back/RConn2
  Left Leg Back/RConn2 -- Left hip back to torso/RConn1
  Right hip front to torso/LConn1 -- R/RConn1 -- Right hip back to torso/LConn1 -- Left hip back to torso/LConn1 -- Torso/RConn1 -- Left hip front to torso/LConn1
  PS-Simulink Converter/LConn1 -- Qquat/RConn1
  Upper leg RF/RConn1 -- "Right Leg Front "/LConn1
  Lower leg RF/RConn1 -- "Right Leg Front "/LConn2
  "Right Leg Front "/LConn3 -- Foot RF/RConn1
  Foot LF/RConn1 -- "Left Leg Front "/LConn3
  Upper leg LF/RConn1 -- "Left Leg Front "/LConn1
  Lower leg LF/RConn1 -- "Left Leg Front "/LConn2
  Upper leg RB/RConn1 -- Right Leg Back/LConn1
  Lower leg RB/RConn1 -- Right Leg Back/LConn2
  Foot RB/RConn1 -- Right Leg Back/LConn3
  Lower leg LB/RConn1 -- Left Leg Back/LConn2
  Left Leg Back/LConn1 -- Upper leg LB/RConn1
  w_torso/RConn1 -- PS-Simulink Converter1/LConn1
  Left Leg Back/LConn3 -- Foot LB/RConn1

== system final_quadruped_230622/Signal Builder ==
  Demux : Demux  Tag=STV Demux  Outputs=1
      settings: DisplayOption=none
  FromWs : FromWorkspace  Tag=STV FromWs  VariableName=tuvar
      SigBuilderData=|
      | common.afterFinalStr = 'Extrapolate'
      | common.sampleTime = 0
      | dataSet.timeRange = [0 10]
      | dataSet.name = 'Group 1'
      | sbobj.Groups.Name = 'Group 1'
      | sbobj.Groups.Signals.Name = 'Signal 1'
      | sbobj.Groups.Signals.XData = [0 0.2 0.2 0.4 4 6 10]
      | sbobj.Groups.Signals.YData = [20 20 0 0 0 0 0]
  Signal 1 : Outport  Tag=STV Outport
  wires:
  Demux/1 -> Signal 1/1
  FromWs/1 -> Demux/1
